simulink model "SatDinModel_3_TES_RW_OL"  (Simulink 7.7)
settings: Solver=ode45  StartTime=0.0  StopTime=40  FixedStep=1  RelTol=1e-3
undefined symbols (not defined in the file or in its folder): coe2rv, e0_0, e1_0, e2_0, e3_0, pm_0, rv2OrbFrame, sigbuilder_block, Vm_0, xme_0
libraries: aerolibtransform2 x8, aerolibconvert2 x8, aerolibutil x3, simulink x2, aerolibanimutils x1, aerolibanim x1, vrlib x1
settings Model: Creator=Ridanto  LastModifiedBy=Ridanto  BufferReuse=off
settings OptimizationCC: BufferReuse=off  InitFltsAndDblsToZero=on
settings DebuggingCC: SaveWithParameterizedLinksMsg=none  SignalResolutionControl=TryResolveAllWithWarning  MultiTaskDSMMsg=warning  MultiTaskCondExecSysMsg=none  StrictBusMsg=Warning
settings SFSimCC: SimParseCustomCode=off
settings RTWCC: IncludeERTFirstTime=on
settings GRTTargetCC: TargetFcnLib=ansi_tfl_tmw.mat

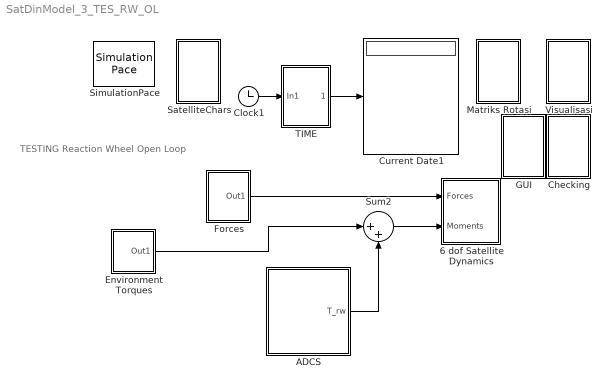
== system SatDinModel_3_TES_RW_OL ==
  note: TESTING
      | Reaction Wheel Open Loop
  6 dof Satellite Dynamics : Subsystem
  ADCS : Subsystem
  Checking : Subsystem
  Clock1 : Clock
      settings: Decimation=10
  Current Date1 : Display
  Environment Torques : Subsystem
  Forces : Subsystem
  GUI : Subsystem
  Matriks Rotasi : Subsystem
  SatelliteChars : Subsystem
  SimulationPace : aerolibanimutils/Simulation Pace  SimulationPace=60  SleepMode=MATLAB Thread  OutputPaceError=off  SampleTime=1/30
      settings: AttributesFormatString=%<SimulationPace> sec/sec
  Sum2 : Sum  Inputs=|++
  TIME : Subsystem
  Visualisasi : Subsystem
  wires:
  Clock1/1 -> TIME/1(In1)
  TIME/1(Out1) -> Current Date1/1
  Environment Torques/1(Out1) -> Sum2/1
  Sum2/1 -> 6 dof Satellite Dynamics/2(Moments)
  Forces/1(Out1) -> 6 dof Satellite Dynamics/1(Forces)
  ADCS/1(T_rw) -> Sum2/2

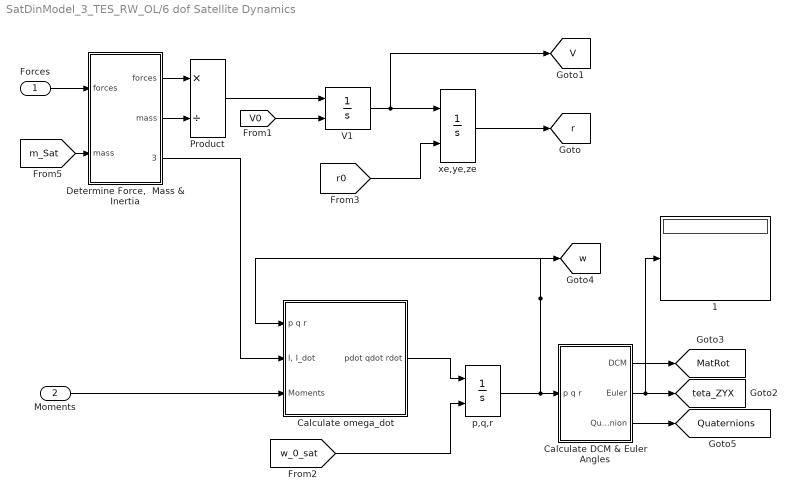
== system SatDinModel_3_TES_RW_OL/6 dof Satellite Dynamics ==
  Forces : Inport
  Moments : Inport  Port=2
  1 : Display
  Calculate DCM & Euler Angles : Subsystem  AncestorBlock=aerolib6dofsys/DCM & Euler Angles (Quaternion)
      mask Type: DCM & Euler Angles (Quaternion)
  Calculate omega_dot : Subsystem  AncestorBlock=aerolib6dofsys/Calculate omega_dot
  "Determine Force,  Mass & Inertia" : Subsystem  AncestorBlock=aerolib6dofsys/Mass & Inertia (fixed)
      mask Type: Mass & Inertia (fixed)
  Product : Product  Inputs=*/  SaturateOnIntegerOverflow=on  OutDataTypeStr=Inherit: Same as first input
  V1 : Integrator  InitialConditionSource=external  InitialCondition=convvel(Vm_0,'m/s','m/s')
  "p,q,r " : Integrator  InitialConditionSource=external  InitialCondition=pm_0
  xe,ye,ze : Integrator  InitialConditionSource=external  InitialCondition=xme_0
  tag scope: MatRot=global, Quaternions=global, V=global, r=global, teta_ZYX=global, w=global
  wires:
  "Determine Force,  Mass & Inertia"/1("forces ") -> Product/1
  Calculate omega_dot/1(pdot qdot rdot) -> "p,q,r "/1
  "Determine Force,  Mass & Inertia"/2(mass) -> Product/2
  Calculate DCM & Euler Angles/1(DCM) -> [MatRot]
  Product/1 -> V1/1
  Forces/1 -> "Determine Force,  Mass & Inertia"/1(forces)
  Moments/1 -> Calculate omega_dot/3(Moments)
  "p,q,r "/1 -> Calculate omega_dot/1(p q r), Calculate DCM & Euler Angles/1(p q r), [w]
  xe,ye,ze/1 -> [r]
  Calculate DCM & Euler Angles/2(Euler) -> [teta_ZYX], 1/1
  "Determine Force,  Mass & Inertia"/3("inertia, 0") -> Calculate omega_dot/2("I, I_dot")
  [w_0_sat] -> "p,q,r "/2
  [r0] -> xe,ye,ze/2
  Calculate DCM & Euler Angles/3(Quaternion) -> [Quaternions]
  [m_Sat] -> "Determine Force,  Mass & Inertia"/2("mass ")
  [V0] -> V1/2
  V1/1 -> xe,ye,ze/1, [V]

== system SatDinModel_3_TES_RW_OL/ADCS ==
  Mux : Mux  Inputs=3
  RW_3_Axis : Subsystem
  Signal Builder : Subsystem  Tag=STV Subsys  LoadFcn=sigbuilder_block('load');  StartFcn=sigbuilder_block('start');  StopFcn=sigbuilder_block('stop');  ClipboardFcn=sigbuilder_block('clipboard');  mask(Sigbuilder block){}
      mask help: Create and generate interchangeable groups of signals whose waveforms are piecewise linear.
      mask init:
      | if ~strcmp(get_param(bdroot(gcbh),'SimulationStatus'),'stopped') tuvar = sigbuilder_block('maskInit'); end
      settings: CopyFcn=sigbuilder_block('copy');  DeleteFcn=sigbuilder_block('delete');  ModelCloseFcn=sigbuilder_block('modelClose');  PreSaveFcn=sigbuilder_block('preSave');  NameChangeFcn=sigbuilder_block('namechange');  OpenFcn=sigbuilder_block('open',[437.25 96 550.5 394.5 ]);  CloseFcn=sigbuilder_block('close');
      mask Display: plot(0, 0, 100, 100,[2, 2, 32, 32, 2], [68, 8, 8, 68, 68],[32, 2], [38, 38], [32, 19, 2],[53, 60, 44], [32, 17, 17, 2],[16, 16, 31, 31]);txt = getActiveGroup(gcbh);text(2, 100, txt,'verticalAlignment', 'top');
  w_rw : Scope
      settings: SaveName=ScopeData6
  T_rw : Outport
  tag scope: H_rw=global, w_rw=global
  wires:
  RW_3_Axis/1(T_rw) -> T_rw/1
  RW_3_Axis/2(w_rw) -> [w_rw], w_rw/1
  RW_3_Axis/3(H_rw) -> [H_rw]
  Mux/1 -> RW_3_Axis/1(T_c)
  Signal Builder/1(Signal 1) -> Mux/1
  Signal Builder/2(Signal 5) -> Mux/2
  Signal Builder/3(Signal 6) -> Mux/3

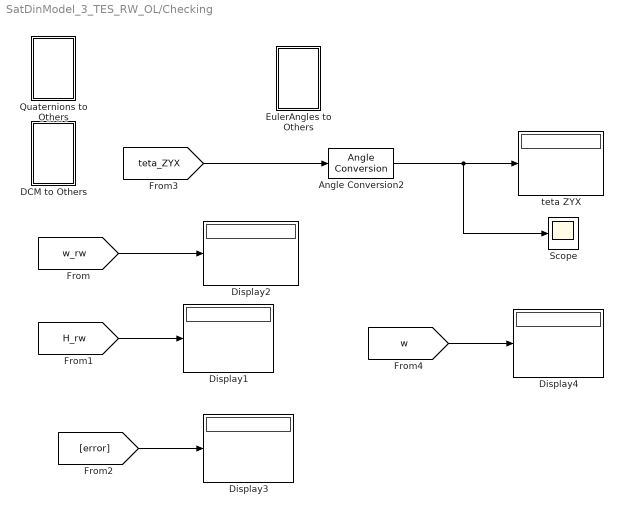
== system SatDinModel_3_TES_RW_OL/Checking ==
  Angle Conversion2 : aerolibconvert2/Angle Conversion  SystemSampleTime=-1  IU=rad  OU=deg
  DCM to Others : Subsystem
  Display{1..4} (4 alike) : Display
  EulerAngles to Others : Subsystem
  Quaternions to Others : Subsystem
  Scope : Scope
      settings: YMin=0  YMax=0.00275
  teta ZYX : Display
  wires:
  [H_rw] -> Display1/1
  [w_rw] -> Display2/1
  [error] -> Display3/1
  [teta_ZYX] -> Angle Conversion2/1
  [w] -> Display4/1
  Angle Conversion2/1 -> teta ZYX/1, Scope/1

== system SatDinModel_3_TES_RW_OL/Environment Torques ==
  "Env Torque, Nm" : Subsystem  Tag=STV Subsys  LoadFcn=sigbuilder_block('load');  StartFcn=sigbuilder_block('start');  StopFcn=sigbuilder_block('stop');  ClipboardFcn=sigbuilder_block('clipboard');  mask(Sigbuilder block){}
      mask help: Create and generate interchangeable groups of signals whose waveforms are piecewise linear.
      mask init:
      | if ~strcmp(get_param(bdroot(gcbh),'SimulationStatus'),'stopped') tuvar = sigbuilder_block('maskInit'); end
      settings: CopyFcn=sigbuilder_block('copy');  DeleteFcn=sigbuilder_block('delete');  ModelCloseFcn=sigbuilder_block('modelClose');  PreSaveFcn=sigbuilder_block('preSave');  NameChangeFcn=sigbuilder_block('namechange');  OpenFcn=sigbuilder_block('open',[437.25 96 550.5 394.5 ]);  CloseFcn=sigbuilder_block('close');
      mask Display: plot(0,0,100,100,[10,10,40,40,10],[80,20,20,80,80],[40,10],[50,50], [40,27,10],[65,72,56],[40,25,25,10],[28,28,43,43]);
  Manual Switch : simulink/Signal Routing/Manual Switch  SystemSampleTime=-1  sw=1  action=0  varsize=off
  Mux : Mux  Inputs=3
  No Torque : Constant  Value=[0 0 0]
  Typical LEO SSO : Gain  Gain=4.586e-5
  xxx : Constant  Value=0
  Out1 : Outport
  wires:
  xxx/1 -> Mux/2, Mux/3
  Mux/1 -> Manual Switch/2
  No Torque/1 -> Manual Switch/1
  Manual Switch/1 -> Out1/1
  "Env Torque, Nm"/1(Signal 1) -> Typical LEO SSO/1
  Typical LEO SSO/1 -> Mux/1

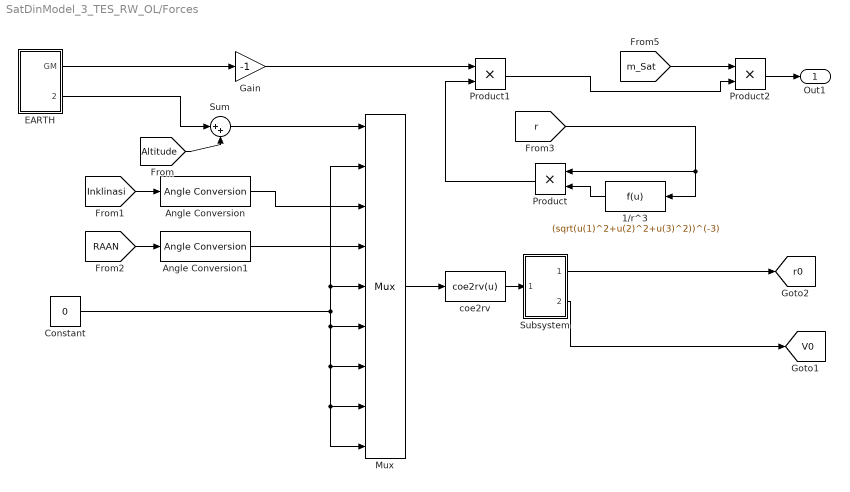
== system SatDinModel_3_TES_RW_OL/Forces ==
  1/r^3 : Fcn  Expr=(sqrt(u(1)^2+u(2)^2+u(3)^2))^(-3)
  Angle Conversion : aerolibconvert2/Angle Conversion  SystemSampleTime=-1  IU=deg  OU=rad
  Angle Conversion1 : aerolibconvert2/Angle Conversion  SystemSampleTime=-1  IU=deg  OU=rad
  Constant : Constant  Value=0
  EARTH : Subsystem
  Gain : Gain  Gain=-1
  Mux : Mux  Inputs=9
  Product : Product  RndMeth=Zero
  Product1 : Product  RndMeth=Zero
  Product2 : Product  RndMeth=Zero
  Subsystem : Subsystem
  Sum : Sum  Inputs=|++
  coe2rv : MATLABFcn  MATLABFcn=coe2rv(u)
  Out1 : Outport
  tag scope: V0=global, r0=global
  wires:
  EARTH/1(GM) -> Gain/1
  EARTH/2(Radius) -> Sum/1
  Angle Conversion/1 -> Mux/3
  Sum/1 -> Mux/1
  Angle Conversion1/1 -> Mux/4
  Mux/1 -> coe2rv/1
  coe2rv/1 -> Subsystem/1(In1)
  Constant/1 -> Mux/2, Mux/5, Mux/6, Mux/7, Mux/8, Mux/9
  [Altitude] -> Sum/2
  [Inklinasi] -> Angle Conversion/1
  [RAAN] -> Angle Conversion1/1
  Subsystem/1(Out1) -> [r0]
  1/r^3/1 -> Product/2
  Product/1 -> Product1/2
  Gain/1 -> Product1/1
  Product1/1 -> Product2/2
  [r] -> 1/r^3/1, Product/1
  [m_Sat] -> Product2/1
  Product2/1 -> Out1/1
  Subsystem/2(Out2) -> [V0]

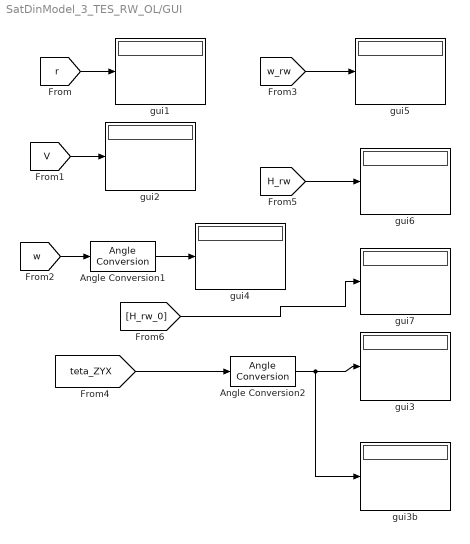
== system SatDinModel_3_TES_RW_OL/GUI ==
  Angle Conversion1 : aerolibconvert2/Angle Conversion  SystemSampleTime=-1  IU=rad  OU=deg
  Angle Conversion2 : aerolibconvert2/Angle Conversion  SystemSampleTime=-1  IU=rad  OU=deg
  gui{1..7} (7 alike) : Display
  gui3b : Display
  wires:
  [r] -> gui1/1
  [V] -> gui2/1
  Angle Conversion1/1 -> gui4/1
  [w] -> Angle Conversion1/1
  [teta_ZYX] -> Angle Conversion2/1
  Angle Conversion2/1 -> gui3/1, gui3b/1
  [w_rw] -> gui5/1
  [H_rw] -> gui6/1
  [H_rw_0] -> gui7/1

== system SatDinModel_3_TES_RW_OL/Matriks Rotasi ==
  Math Function : Math  Operator=transpose  SaturateOnIntegerOverflow=on
  Matriks Rotasi Benda-Inersial : Display
  Matriks Rotasi Benda-Orbital : Display
  Matriks Rotasi Orbital-Inersial : Display
  Mux1 : Mux  Inputs=2
  Product : Product  Multiplication=Matrix(*)  RndMeth=Zero
  rv2OrbFrame : MATLABFcn  MATLABFcn=rv2OrbFrame(u)  Output1D=off
  tag scope: R_oi=global
  wires:
  [r] -> Mux1/1
  [V] -> Mux1/2
  Mux1/1 -> rv2OrbFrame/1
  rv2OrbFrame/1 -> Matriks Rotasi Orbital-Inersial/1, Math Function/1, [R_oi]
  [MatRot] -> Matriks Rotasi Benda-Inersial/1, Product/1
  Math Function/1 -> Product/2
  Product/1 -> Matriks Rotasi Benda-Orbital/1

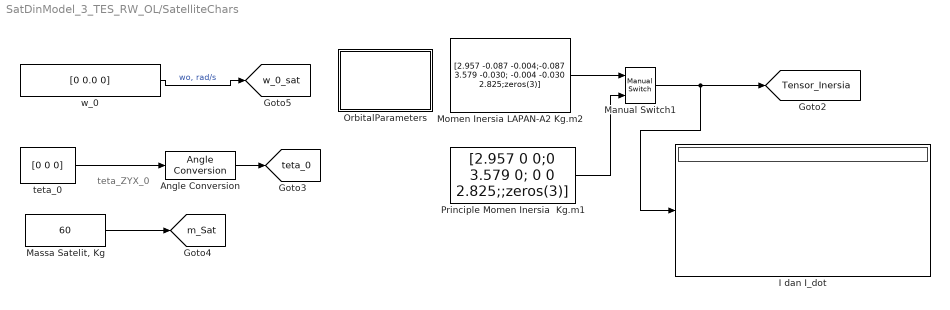
== system SatDinModel_3_TES_RW_OL/SatelliteChars ==
  note: teta_ZYX_0
  Angle Conversion : aerolibconvert2/Angle Conversion  SystemSampleTime=-1  IU=deg  OU=rad
  I dan I_dot : Display
  Manual Switch1 : simulink/Signal Routing/Manual Switch  SystemSampleTime=-1  sw=1  action=0  varsize=off
  "Massa Satelit, Kg" : Constant  Value=60
  Momen Inersia LAPAN-A2 Kg.m2 : Constant  Value=[2.957 -0.087 -0.004;-0.087 3.579 -0.030; -0.004 -0.030 2.825;zeros(3)]
  OrbitalParameters : Subsystem
  Principle Momen Inersia  Kg.m1 : Constant  Value=[2.957 0 0;0 3.579 0; 0 0 2.825;;zeros(3)]
  teta_0 : Constant  Value=[0 0 0]
  w_0 : Constant  Value=[0 0.0 0]
  tag scope: Tensor_Inersia=global, m_Sat=global, teta_0=global, w_0_sat=global
  wires:
  teta_0/1 -> Angle Conversion/1
  "Massa Satelit, Kg"/1 -> [m_Sat]
  Angle Conversion/1 -> [teta_0]
  Principle Momen Inersia  Kg.m1/1 -> Manual Switch1/2
  Momen Inersia LAPAN-A2 Kg.m2/1 -> Manual Switch1/1
  Manual Switch1/1 -> [Tensor_Inersia], I dan I_dot/1
  w_0/1 -> [w_0_sat]  "wo, rad/s"

== system SatDinModel_3_TES_RW_OL/TIME ==
  In1 : Inport
  Embedded MATLAB Function : Stateflow chart  TreatAsAtomicUnit=on
  JD : Display
  Sum1 : Sum  Inputs=|++
  day2second : Gain  Gain=1/3600/24
  detik : Display
  Out1 : Outport
  wires:
  In1/1 -> detik/1, day2second/1
  day2second/1 -> Sum1/1
  Sum1/1 -> Embedded MATLAB Function/1(jd), JD/1
  Embedded MATLAB Function/1(y) -> Out1/1
  [Mulai] -> Sum1/2

== system SatDinModel_3_TES_RW_OL/Visualisasi ==
  6DoF Animation : aerolibanim/6DoF Animation  SystemSampleTime=-1  u1=[-10000 10000 -10000 10000 -10000 10000]  u2=2  u3=2000  u4=[0 0 0]  u5=Fixed position  u6=[60000 120000 60000]  u7=10  u8=on
      link override Animation S-Function: FunctionName=sSATanim3
  Display : Display
  Gain : Gain  Gain=1/500
  Selector : Selector  InputPortWidth=3  IndexOptions=Index vector (dialog)  Indices=[3 2 1]  OutputSizes=1
  VR Sink1 : vrlib/VR Sink  SampleTime=20  ViewEnable=on  RemoteChange=off  RemoteView=on  FieldsWritten=satelit.rotation.4.1.1.double#satelit.translation.3.1.1.double  WorldFileName=vrattsat.WRL  AutoView=off  VideoDimensions=[]  FigureProperties={}
  wires:
  [teta_ZYX] -> Selector/1
  [r] -> 6DoF Animation/1, Display/1, Gain/1
  Selector/1 -> 6DoF Animation/2
  [Quaternions] -> VR Sink1/1
  Gain/1 -> VR Sink1/2

== system SatDinModel_3_TES_RW_OL/6 dof Satellite Dynamics/Calculate DCM & Euler Angles ==
  p q r : Inport
  Quaternions to  Direction Cosine Matrix : aerolibtransform2/Quaternions to  Direction Cosine Matrix  SystemSampleTime=-1
  Quaternions to Rotation Angles : aerolibtransform2/Quaternions to Rotation Angles  SystemSampleTime=-1  rotationOrder=ZYX
  Rotation Angles to Quaternions : aerolibtransform2/Rotation Angles to Quaternions  SystemSampleTime=-1  rotationOrder=ZYX
  q0 q1 q2 q3 : Integrator  InitialConditionSource=external  InitialCondition=[e0_0 e1_0 e2_0 e3_0]
  qdot : Subsystem
  DCM : Outport
  Euler : Outport  Port=2
  Quaternion : Outport  Port=3
  wires:
  Quaternions to Rotation Angles/1 -> Euler/1
  Quaternions to  Direction Cosine Matrix/1 -> DCM/1
  p q r/1 -> qdot/1(p q r)
  [teta_0] -> Rotation Angles to Quaternions/1
  Rotation Angles to Quaternions/1 -> q0 q1 q2 q3/2
  q0 q1 q2 q3/1 -> Quaternions to Rotation Angles/1, qdot/2(q0 q1 q2 q3), Quaternions to  Direction Cosine Matrix/1, Quaternion/1
  qdot/1(qdot) -> q0 q1 q2 q3/1

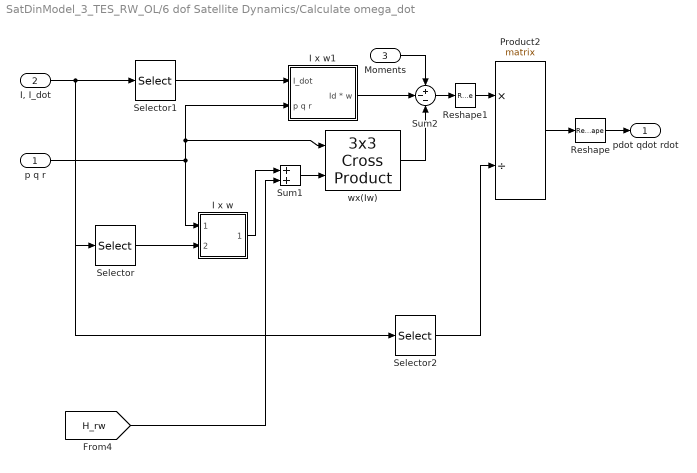
== system SatDinModel_3_TES_RW_OL/6 dof Satellite Dynamics/Calculate omega_dot ==
  p q r : Inport
  "I, I_dot" : Inport  Port=2
  Moments : Inport  Port=3
  I x w : Subsystem
  I x w1 : Subsystem
  Product2 : Product  Inputs=*/  Multiplication=Matrix(*)  SaturateOnIntegerOverflow=on  OutDataTypeStr=Inherit: Same as first input
  Reshape : Reshape
  Reshape1 : Reshape  OutputDimensionality=Row vector (2-D)
  Selector : Selector  NumberOfDimensions=2  InputPortWidth=2  IndexOptions=Index vector (dialog),Select all  Indices=1:3,-1  OutputSizes=1
  Selector1 : Selector  NumberOfDimensions=2  InputPortWidth=2  IndexOptions=Index vector (dialog),Select all  Indices=4:6,-1  OutputSizes=1
  Selector2 : Selector  NumberOfDimensions=2  InputPortWidth=2  IndexOptions=Index vector (dialog),Select all  Indices=1:3,-1  OutputSizes=1
  Sum1 : Sum  SaturateOnIntegerOverflow=on
  Sum2 : Sum  Inputs=+--  SaturateOnIntegerOverflow=on
  wx(Iw) : aerolibutil/3x3 Cross Product  SystemSampleTime=-1
  pdot qdot rdot : Outport
  wires:
  Reshape1/1 -> Product2/1
  wx(Iw)/1 -> Sum2/3
  Selector1/1 -> I x w1/1(I_dot)
  I x w1/1(Id * w) -> Sum2/2
  Moments/1 -> Sum2/1
  Sum2/1 -> Reshape1/1
  Product2/1 -> Reshape/1
  p q r/1 -> I x w1/2(p q r), wx(Iw)/1, I x w/1(p q r)
  "I, I_dot"/1 -> Selector1/1, Selector2/1, Selector/1
  Selector2/1 -> Product2/2
  Selector/1 -> I x w/2(Inertia)
  Reshape/1 -> pdot qdot rdot/1
  Sum1/1 -> wx(Iw)/2
  I x w/1(I * w) -> Sum1/1
  [H_rw] -> Sum1/2

== system SatDinModel_3_TES_RW_OL/6 dof Satellite Dynamics/Determine Force,  Mass & Inertia ==
  forces : Inport
  "mass " : Inport  Port=2
  "forces " : Outport
  mass : Outport  Port=2
  "inertia, 0" : Outport  Port=3
  wires:
  forces/1 -> "forces "/1
  [Tensor_Inersia] -> "inertia, 0"/1
  "mass "/1 -> mass/1

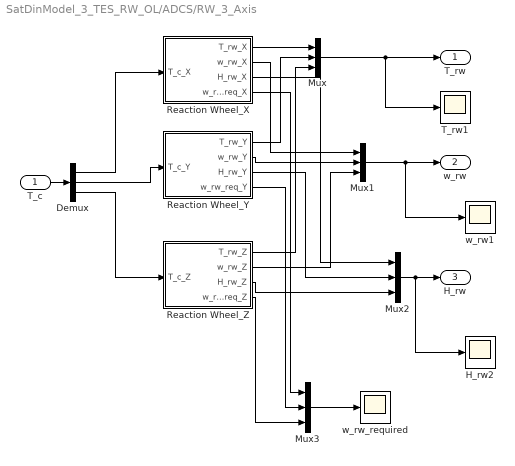
== system SatDinModel_3_TES_RW_OL/ADCS/RW_3_Axis ==
  T_c : Inport
  Demux : Demux  Outputs=3
  H_rw2 : Scope
      settings: SaveName=ScopeData3
  Mux{,1..3} (4 alike) : Mux  Inputs=3
  Reaction Wheel_X : Subsystem
  Reaction Wheel_Y : Subsystem
  Reaction Wheel_Z : Subsystem
  T_rw1 : Scope
      settings: SaveName=ScopeData10
  w_rw1 : Scope
  w_rw_required : Scope
      settings: SaveName=ScopeData2
  T_rw : Outport
  w_rw : Outport  Port=2
  H_rw : Outport  Port=3
  wires:
  Reaction Wheel_Y/1(T_rw_Y) -> Mux/2
  T_c/1 -> Demux/1
  Demux/1 -> Reaction Wheel_X/1(T_c_X)
  Demux/2 -> Reaction Wheel_Y/1(T_c_Y)
  Demux/3 -> Reaction Wheel_Z/1(T_c_Z)
  Reaction Wheel_X/1(T_rw_X) -> Mux/1
  Reaction Wheel_Z/1(T_rw_Z) -> Mux/3
  Mux/1 -> T_rw/1, T_rw1/1
  Mux1/1 -> w_rw/1, w_rw1/1
  Reaction Wheel_Y/2(w_rw_Y) -> Mux1/2
  Reaction Wheel_X/2(w_rw_X) -> Mux1/1
  Reaction Wheel_Z/2(w_rw_Z) -> Mux1/3
  Mux2/1 -> H_rw/1, H_rw2/1
  Reaction Wheel_Z/3(H_rw_Z) -> Mux2/3
  Reaction Wheel_X/3(H_rw_X) -> Mux2/1
  Reaction Wheel_Y/3(H_rw_Y) -> Mux2/2
  Mux3/1 -> w_rw_required/1
  Reaction Wheel_X/4(w_rw_req_X) -> Mux3/1
  Reaction Wheel_Y/4(w_rw_req_Y) -> Mux3/2
  Reaction Wheel_Z/4(w_rw_req_Z) -> Mux3/3

== system SatDinModel_3_TES_RW_OL/ADCS/Signal Builder ==
  Demux : Demux  Tag=STV Demux  Outputs=3
  FromWs : FromWorkspace  Tag=STV FromWs  VariableName=tuvar  SampleTime=0  SigBuilderData=DataTag0  VnvData=DataTag1
      SigBuilderData=|
      | common.afterFinalStr = 'Extrapolate'
      | common.sampleTime = 0
      | dataSet.timeRange = [0 10]
      | dataSet.name = 'Group 1'
      | sbobj.Groups.Name = 'Group 1'
      | sbobj.Groups.Signals(1).Name = 'Signal 1'
      | sbobj.Groups.Signals(1).XData = [0 4 4 5.04 5.04 10]
      | sbobj.Groups.Signals(1).YData = [0 0 0.1 0.1 0 0]
      | sbobj.Groups.Signals(2).Name = 'Signal 5'
      | sbobj.Groups.Signals(2).XData = [0 4 4 6 6 10]
      | sbobj.Groups.Signals(2).YData = [0 0 0.1 0.1 0 0]
      | sbobj.Groups.Signals(3).Name = 'Signal 6'
      | sbobj.Groups.Signals(3).XData = [0 5 5 7 7 10]
      | sbobj.Groups.Signals(3).YData = [0 0 0.062 0.062 0 0]
  Signal 1 : Outport  Tag=STV Outport
  Signal 5 : Outport  Tag=STV Outport  Port=2
  Signal 6 : Outport  Tag=STV Outport  Port=3
  wires:
  Demux/1 -> Signal 1/1
  FromWs/1 -> Demux/1
  Demux/2 -> Signal 5/1
  Demux/3 -> Signal 6/1

== system SatDinModel_3_TES_RW_OL/Checking/DCM to Others ==
  Angle Conversion : aerolibconvert2/Angle Conversion  SystemSampleTime=-1  IU=rad  OU=deg
  Direction Cosine Matrix  to Quaternions : aerolibtransform2/Direction Cosine Matrix  to Quaternions  SystemSampleTime=-1
  "Quaternions q0, q1, q2, q3" : Display
  Quaternions to Rotation Angles : aerolibtransform2/Quaternions to Rotation Angles  SystemSampleTime=-1  rotationOrder=ZYX
  teta_Euler ZYX : Display
  "teta_Euler ZYX " : Display
  wires:
  Quaternions to Rotation Angles/1 -> teta_Euler ZYX/1, Angle Conversion/1
  Angle Conversion/1 -> "teta_Euler ZYX "/1
  [MatRot] -> Direction Cosine Matrix  to Quaternions/1
  Direction Cosine Matrix  to Quaternions/1 -> "Quaternions q0, q1, q2, q3"/1, Quaternions to Rotation Angles/1

== system SatDinModel_3_TES_RW_OL/Checking/EulerAngles to Others ==
  Direction Cosine Matrix  to Quaternions : aerolibtransform2/Direction Cosine Matrix  to Quaternions  SystemSampleTime=-1
  Matriks Rotasi Benda-Inersial R_bi : Display
  "Quaternions q0, q1, q2, q3" : Display
  teta_ZYX to DCM : Subsystem
  wires:
  [teta_ZYX] -> teta_ZYX to DCM/1(In2)
  Direction Cosine Matrix  to Quaternions/1 -> "Quaternions q0, q1, q2, q3"/1
  teta_ZYX to DCM/1(Out1) -> Matriks Rotasi Benda-Inersial R_bi/1, Direction Cosine Matrix  to Quaternions/1

== system SatDinModel_3_TES_RW_OL/Checking/Quaternions to Others ==
  Angle Conversion : aerolibconvert2/Angle Conversion  SystemSampleTime=-1  IU=rad  OU=deg
  Matriks Rotasi Benda-Inersial R_bi : Display
  Matriks Rotasi Benda-Inersial R_bi _juga : Display
  Quaternions to  Direction Cosine Matrix : aerolibtransform2/Quaternions to  Direction Cosine Matrix  SystemSampleTime=-1
  Quaternions to Rotation Angles : aerolibtransform2/Quaternions to Rotation Angles  SystemSampleTime=-1  rotationOrder=ZYX
  teta_Euler ZYX : Display
  "teta_Euler ZYX " : Display
  teta_ZYX to DCM : Subsystem
  wires:
  Quaternions to Rotation Angles/1 -> teta_Euler ZYX/1, Angle Conversion/1, teta_ZYX to DCM/1(In2)
  teta_ZYX to DCM/1(Out1) -> Matriks Rotasi Benda-Inersial R_bi/1
  Quaternions to  Direction Cosine Matrix/1 -> Matriks Rotasi Benda-Inersial R_bi _juga/1
  Angle Conversion/1 -> "teta_Euler ZYX "/1
  [Quaternions] -> Quaternions to Rotation Angles/1, Quaternions to  Direction Cosine Matrix/1

== system SatDinModel_3_TES_RW_OL/Environment Torques/Env Torque, Nm ==
  Demux : Demux  Tag=STV Demux  Outputs=1
  FromWs : FromWorkspace  Tag=STV FromWs  VariableName=tuvar  SampleTime=0  SigBuilderData=DataTag2  VnvData=DataTag3
      SigBuilderData=|
      | common.afterFinalStr = 'Extrapolate'
      | common.sampleTime = 0
      | dataSet.timeRange = [0 10]
      | dataSet.name = 'Group 1'
      | sbobj.Groups.Name = 'Group 1'
      | sbobj.Groups.Signals.Name = 'Signal 1'
      | sbobj.Groups.Signals.XData = [0 4 4 6 6 10]
      | sbobj.Groups.Signals.YData = [0 0 1 1 0 0]
  Signal 1 : Outport  Tag=STV Outport
  wires:
  Demux/1 -> Signal 1/1
  FromWs/1 -> Demux/1

== system SatDinModel_3_TES_RW_OL/Forces/EARTH ==
  GM Earth : Constant  Value=3.986e5
  Re : Constant  Value=6378
  GM : Outport
  Radius : Outport  Port=2
  wires:
  GM Earth/1 -> GM/1
  Re/1 -> Radius/1

== system SatDinModel_3_TES_RW_OL/Forces/Subsystem ==
  In1 : Inport
  Demux : Demux  Outputs=6
  Mux1 : Mux  Inputs=3
  Mux2 : Mux  Inputs=3
  Out1 : Outport
  Out2 : Outport  Port=2
  wires:
  Demux/1 -> Mux1/1
  Demux/2 -> Mux1/2
  Demux/3 -> Mux1/3
  Demux/4 -> Mux2/1
  Demux/5 -> Mux2/2
  Demux/6 -> Mux2/3
  Mux1/1 -> Out1/1
  In1/1 -> Demux/1
  Mux2/1 -> Out2/1

== system SatDinModel_3_TES_RW_OL/SatelliteChars/OrbitalParameters ==
  Epoch : Constant  Value=735578.8723
  H : Constant  Value=800
  Inclination : Constant  Value=98.7192
  RAAN : Constant  Value=86.1494
  tag scope: Altitude=global, Inklinasi=global, Mulai=global, RAAN=global
  wires:
  H/1 -> [Altitude]
  Inclination/1 -> [Inklinasi]
  RAAN/1 -> [RAAN]
  Epoch/1 -> [Mulai]

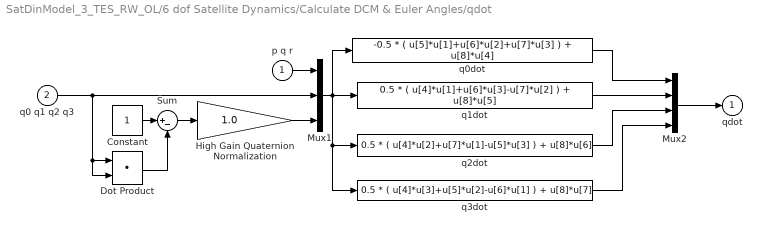
== system SatDinModel_3_TES_RW_OL/6 dof Satellite Dynamics/Calculate DCM & Euler Angles/qdot ==
  p q r : Inport
  q0 q1 q2 q3 : Inport  Port=2
  Constant : Constant
  Dot Product : DotProduct  OutDataTypeStr=Inherit: Inherit via internal rule
  High Gain Quaternion Normalization : Gain  Gain=1.0  SaturateOnIntegerOverflow=on  OutDataTypeStr=Inherit: Same as input  ParamDataTypeStr=Inherit: Same as input
  Mux1 : Mux  Inputs=[3 4 1]
  Mux2 : Mux
  Sum : Sum  Inputs=|+-  SaturateOnIntegerOverflow=on  InputSameDT=on  OutDataTypeStr=Inherit: Same as first input
  q0dot : Fcn  Expr=-0.5 * ( u[5]*u[1]+u[6]*u[2]+u[7]*u[3] ) + u[8]*u[4]
  q1dot : Fcn  Expr=0.5 * ( u[4]*u[1]+u[6]*u[3]-u[7]*u[2] ) + u[8]*u[5]
  q2dot : Fcn  Expr=0.5 * ( u[4]*u[2]+u[7]*u[1]-u[5]*u[3] ) + u[8]*u[6]
  q3dot : Fcn  Expr=0.5 * ( u[4]*u[3]+u[5]*u[2]-u[6]*u[1] ) + u[8]*u[7]
  qdot : Outport  InitialOutput=0
  wires:
  p q r/1 -> Mux1/1
  Dot Product/1 -> Sum/2
  High Gain Quaternion Normalization/1 -> Mux1/3
  Sum/1 -> High Gain Quaternion Normalization/1
  Constant/1 -> Sum/1
  Mux2/1 -> qdot/1
  q0dot/1 -> Mux2/1
  q1dot/1 -> Mux2/2
  q2dot/1 -> Mux2/3
  Mux1/1 -> q2dot/1, q3dot/1, q0dot/1, q1dot/1
  q3dot/1 -> Mux2/4
  q0 q1 q2 q3/1 -> Dot Product/1, Dot Product/2, Mux1/2

== system SatDinModel_3_TES_RW_OL/6 dof Satellite Dynamics/Calculate omega_dot/I x w ==
  p q r : Inport
  Inertia : Inport  Port=2
  Product : Product  Multiplication=Matrix(*)  SaturateOnIntegerOverflow=on  InputSameDT=on  OutDataTypeStr=Inherit: Same as first input
  Reshape1 : Reshape  OutputDimensionality=Column vector (2-D)
  Reshape2 : Reshape
  I * w : Outport
  wires:
  Reshape2/1 -> I * w/1
  Reshape1/1 -> Product/2
  p q r/1 -> Reshape1/1
  Inertia/1 -> Product/1
  Product/1 -> Reshape2/1

== system SatDinModel_3_TES_RW_OL/6 dof Satellite Dynamics/Calculate omega_dot/I x w1 ==
  I_dot : Inport
  p q r : Inport  Port=2
  Product : Product  Multiplication=Matrix(*)  SaturateOnIntegerOverflow=on  InputSameDT=on  OutDataTypeStr=Inherit: Same as first input
  Reshape1 : Reshape  OutputDimensionality=Column vector (2-D)
  Reshape2 : Reshape
  Id * w : Outport
  wires:
  Reshape2/1 -> Id * w/1
  Reshape1/1 -> Product/2
  Product/1 -> Reshape2/1
  I_dot/1 -> Product/1
  p q r/1 -> Reshape1/1

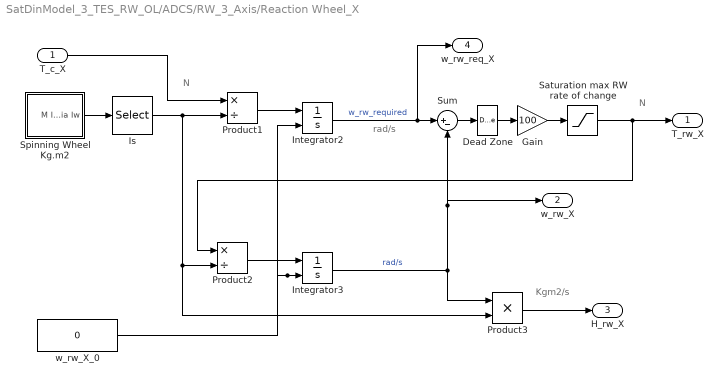
== system SatDinModel_3_TES_RW_OL/ADCS/RW_3_Axis/Reaction Wheel_X ==
  note: rad/s
  note: N
  note: N
  note: Kgm2/s
  T_c_X : Inport
  Dead Zone : DeadZone  SaturateOnIntegerOverflow=on
  Gain : Gain  Gain=100
  Integrator2 : Integrator  InitialConditionSource=external
  Integrator3 : Integrator  InitialConditionSource=external
  Is : Selector  InputPortWidth=3  IndexOptions=Index vector (dialog)  Indices=[1]  OutputSizes=1
  Product1 : Product  Inputs=*/  RndMeth=Zero
  Product2 : Product  Inputs=*/  RndMeth=Zero
  Product3 : Product  RndMeth=Zero
  "Saturation max RW rate of change " : Saturate  UpperLimit=0.0075  LowerLimit=-0.0075
  Spinning Wheel Kg.m2 : Subsystem  mask{D=0.1, t=0.01, rho=5000}
      mask prompts: D "diameter"; t "tebal"; rho "density"
  Sum : Sum  Inputs=|+-
  w_rw_X_0 : Constant  Value=0
  T_rw_X : Outport
  w_rw_X : Outport  Port=2
  H_rw_X : Outport  Port=3
  w_rw_req_X : Outport  Port=4
  wires:
  T_c_X/1 -> Product1/1
  Is/1 -> Product1/2, Product2/2, Product3/2
  Product1/1 -> Integrator2/1
  w_rw_X_0/1 -> Integrator2/2, Integrator3/2
  Integrator2/1 -> Sum/1, w_rw_req_X/1  "w_rw_required"
  Integrator3/1 -> Sum/2, w_rw_X/1, Product3/1  "rad/s"
  Sum/1 -> Dead Zone/1
  Gain/1 -> "Saturation max RW rate of change "/1
  Product2/1 -> Integrator3/1
  "Saturation max RW rate of change "/1 -> Product2/1, T_rw_X/1
  Spinning Wheel Kg.m2/1(M Inertia Iw) -> Is/1
  Product3/1 -> H_rw_X/1
  Dead Zone/1 -> Gain/1

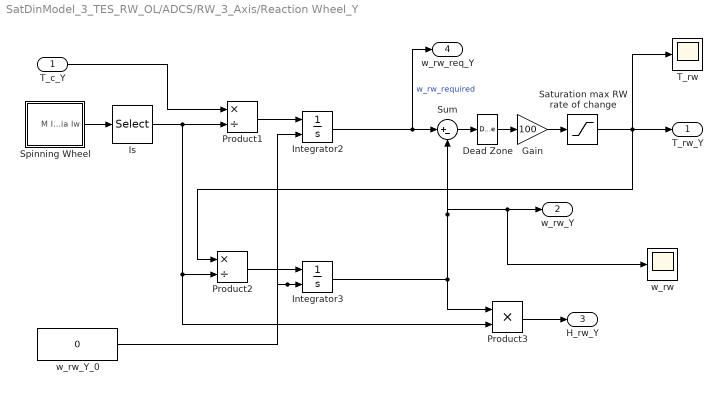
== system SatDinModel_3_TES_RW_OL/ADCS/RW_3_Axis/Reaction Wheel_Y ==
  T_c_Y : Inport
  Dead Zone : DeadZone  SaturateOnIntegerOverflow=on
  Gain : Gain  Gain=100
  Integrator2 : Integrator  InitialConditionSource=external
  Integrator3 : Integrator  InitialConditionSource=external
  Is : Selector  InputPortWidth=3  IndexOptions=Index vector (dialog)  Indices=[1]  OutputSizes=1
  Product1 : Product  Inputs=*/  RndMeth=Zero
  Product2 : Product  Inputs=*/  RndMeth=Zero
  Product3 : Product  RndMeth=Zero
  "Saturation max RW rate of change " : Saturate  UpperLimit=0.0075  LowerLimit=-0.0075
  Spinning Wheel : Subsystem  mask{D=0.1, t=0.01, rho=2850}
      mask prompts: D "diameter"; t "tebal"; rho "density"
  Sum : Sum  Inputs=|+-
  T_rw : Scope
      settings: SaveName=ScopeData11
  w_rw : Scope
      settings: SaveName=ScopeData12
  w_rw_Y_0 : Constant  Value=0
  T_rw_Y : Outport
  w_rw_Y : Outport  Port=2
  H_rw_Y : Outport  Port=3
  w_rw_req_Y : Outport  Port=4
  wires:
  T_c_Y/1 -> Product1/1
  Is/1 -> Product1/2, Product2/2, Product3/2
  Product1/1 -> Integrator2/1
  w_rw_Y_0/1 -> Integrator2/2, Integrator3/2
  Integrator2/1 -> Sum/1, w_rw_req_Y/1  "w_rw_required"
  Integrator3/1 -> Sum/2, w_rw_Y/1, w_rw/1, Product3/1
  Sum/1 -> Dead Zone/1
  Gain/1 -> "Saturation max RW rate of change "/1
  Product2/1 -> Integrator3/1
  "Saturation max RW rate of change "/1 -> Product2/1, T_rw_Y/1, T_rw/1
  Spinning Wheel/1(M Inertia Iw) -> Is/1
  Product3/1 -> H_rw_Y/1
  Dead Zone/1 -> Gain/1

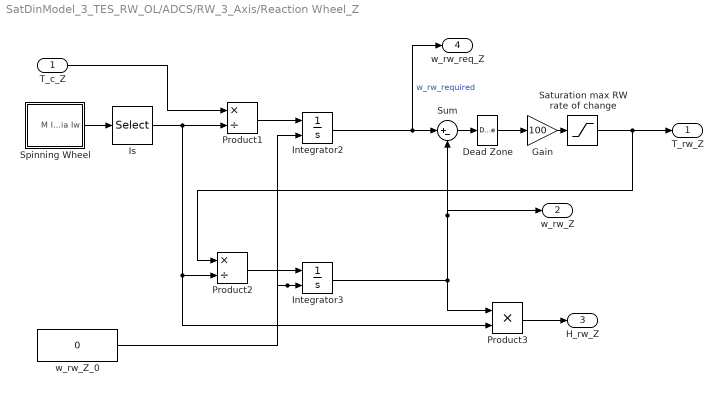
== system SatDinModel_3_TES_RW_OL/ADCS/RW_3_Axis/Reaction Wheel_Z ==
  T_c_Z : Inport
  Dead Zone : DeadZone  SaturateOnIntegerOverflow=on
  Gain : Gain  Gain=100
  Integrator2 : Integrator  InitialConditionSource=external
  Integrator3 : Integrator  InitialConditionSource=external
  Is : Selector  InputPortWidth=3  IndexOptions=Index vector (dialog)  Indices=[1]  OutputSizes=1
  Product1 : Product  Inputs=*/  RndMeth=Zero
  Product2 : Product  Inputs=*/  RndMeth=Zero
  Product3 : Product  RndMeth=Zero
  "Saturation max RW rate of change " : Saturate  UpperLimit=0.0075  LowerLimit=-0.0075
  Spinning Wheel : Subsystem  mask{D=0.1, t=0.01, rho=2850}
      mask prompts: D "diameter"; t "tebal"; rho "density"
  Sum : Sum  Inputs=|+-
  w_rw_Z_0 : Constant  Value=0
  T_rw_Z : Outport
  w_rw_Z : Outport  Port=2
  H_rw_Z : Outport  Port=3
  w_rw_req_Z : Outport  Port=4
  wires:
  T_c_Z/1 -> Product1/1
  Is/1 -> Product1/2, Product2/2, Product3/2
  Product1/1 -> Integrator2/1
  w_rw_Z_0/1 -> Integrator2/2, Integrator3/2
  Integrator2/1 -> Sum/1, w_rw_req_Z/1  "w_rw_required"
  Integrator3/1 -> Sum/2, w_rw_Z/1, Product3/1
  Sum/1 -> Dead Zone/1
  Gain/1 -> "Saturation max RW rate of change "/1
  Product2/1 -> Integrator3/1
  "Saturation max RW rate of change "/1 -> Product2/1, T_rw_Z/1
  Spinning Wheel/1(M Inertia Iw) -> Is/1
  Product3/1 -> H_rw_Z/1
  Dead Zone/1 -> Gain/1

== system SatDinModel_3_TES_RW_OL/Checking/EulerAngles to Others/teta_ZYX to DCM ==
  In2 : Inport
  Create 3x3 Matrix : aerolibutil/Create 3x3 Matrix  SystemSampleTime=-1
  Fcn : Fcn  Expr=cos(u(2))*cos(u(1))
  Fcn1 : Fcn  Expr=cos(u(2))*sin(u(1))
  Fcn2 : Fcn  Expr=-sin(u(2))
  Fcn3 : Fcn  Expr=-cos(u(3))*sin(u(1))+sin(u(3))*sin(u(2))*cos(u(1))
  Fcn4 : Fcn  Expr=cos(u(3))*cos(u(1))+sin(u(3))*sin(u(2))*sin(u(1))
  Fcn5 : Fcn  Expr=sin(u(3))*cos(u(2))
  Fcn6 : Fcn  Expr=sin(u(3))*sin(u(1))+cos(u(3))*sin(u(2))*cos(u(1))
  Fcn7 : Fcn  Expr=-cos(u(1))*sin(u(3))+cos(u(3))*sin(u(2))*sin(u(1))
  Fcn8 : Fcn  Expr=cos(u(3))*cos(u(2))
  Out1 : Outport
  wires:
  Fcn8/1 -> Create 3x3 Matrix/9
  Fcn7/1 -> Create 3x3 Matrix/8
  Fcn6/1 -> Create 3x3 Matrix/7
  Fcn5/1 -> Create 3x3 Matrix/6
  Fcn4/1 -> Create 3x3 Matrix/5
  Fcn3/1 -> Create 3x3 Matrix/4
  Fcn2/1 -> Create 3x3 Matrix/3
  Fcn1/1 -> Create 3x3 Matrix/2
  Fcn/1 -> Create 3x3 Matrix/1
  In2/1 -> Fcn2/1, Fcn3/1, Fcn4/1, Fcn5/1, Fcn6/1, Fcn7/1, Fcn8/1, Fcn1/1, Fcn/1
  Create 3x3 Matrix/1 -> Out1/1

== system SatDinModel_3_TES_RW_OL/Checking/Quaternions to Others/teta_ZYX to DCM ==
  In2 : Inport
  Create 3x3 Matrix : aerolibutil/Create 3x3 Matrix  SystemSampleTime=-1
  Fcn : Fcn  Expr=cos(u(2))*cos(u(1))
  Fcn1 : Fcn  Expr=cos(u(2))*sin(u(1))
  Fcn2 : Fcn  Expr=-sin(u(2))
  Fcn3 : Fcn  Expr=-cos(u(3))*sin(u(1))+sin(u(3))*sin(u(2))*cos(u(1))
  Fcn4 : Fcn  Expr=cos(u(3))*cos(u(1))+sin(u(3))*sin(u(2))*sin(u(1))
  Fcn5 : Fcn  Expr=sin(u(3))*cos(u(2))
  Fcn6 : Fcn  Expr=sin(u(3))*sin(u(1))+cos(u(3))*sin(u(2))*cos(u(1))
  Fcn7 : Fcn  Expr=-cos(u(1))*sin(u(3))+cos(u(3))*sin(u(2))*sin(u(1))
  Fcn8 : Fcn  Expr=cos(u(3))*cos(u(2))
  Out1 : Outport
  wires:
  Fcn8/1 -> Create 3x3 Matrix/9
  Fcn7/1 -> Create 3x3 Matrix/8
  Fcn6/1 -> Create 3x3 Matrix/7
  Fcn5/1 -> Create 3x3 Matrix/6
  Fcn4/1 -> Create 3x3 Matrix/5
  Fcn3/1 -> Create 3x3 Matrix/4
  Fcn2/1 -> Create 3x3 Matrix/3
  Fcn1/1 -> Create 3x3 Matrix/2
  Fcn/1 -> Create 3x3 Matrix/1
  In2/1 -> Fcn2/1, Fcn3/1, Fcn4/1, Fcn5/1, Fcn6/1, Fcn7/1, Fcn8/1, Fcn1/1, Fcn/1
  Create 3x3 Matrix/1 -> Out1/1

== system SatDinModel_3_TES_RW_OL/ADCS/RW_3_Axis/Reaction Wheel_X/Spinning Wheel Kg.m2 ==
  Demux : Demux  Outputs=3
  Moment of Inertia : MATLABFcn  MATLABFcn=momentofinertia_Wheel  Output1D=off
  Mux : Mux  Inputs=3
  Mux1 : Mux  Inputs=3
  db : Constant  Value=rho  VectorParams1D=off
  diameter : Constant  Value=D  VectorParams1D=off
  tebal : Constant  Value=t  VectorParams1D=off
  M Inertia Iw : Outport
  wires:
  db/1 -> Mux/1
  diameter/1 -> Mux/2
  tebal/1 -> Mux/3
  Mux/1 -> Moment of Inertia/1
  Demux/1 -> Mux1/1
  Demux/2 -> Mux1/2
  Demux/3 -> Mux1/3
  Moment of Inertia/1 -> Demux/1
  Mux1/1 -> M Inertia Iw/1

== system SatDinModel_3_TES_RW_OL/ADCS/RW_3_Axis/Reaction Wheel_Y/Spinning Wheel ==
  Demux : Demux  Outputs=3
  Moment of Inertia : MATLABFcn  MATLABFcn=momentofinertia_Wheel  Output1D=off
  Mux : Mux  Inputs=3
  Mux1 : Mux  Inputs=3
  db : Constant  Value=rho  VectorParams1D=off
  diameter : Constant  Value=D  VectorParams1D=off
  tebal : Constant  Value=t  VectorParams1D=off
  M Inertia Iw : Outport
  wires:
  db/1 -> Mux/1
  diameter/1 -> Mux/2
  tebal/1 -> Mux/3
  Mux/1 -> Moment of Inertia/1
  Demux/1 -> Mux1/1
  Demux/2 -> Mux1/2
  Demux/3 -> Mux1/3
  Moment of Inertia/1 -> Demux/1
  Mux1/1 -> M Inertia Iw/1

== system SatDinModel_3_TES_RW_OL/ADCS/RW_3_Axis/Reaction Wheel_Z/Spinning Wheel ==
  Demux : Demux  Outputs=3
  Moment of Inertia : MATLABFcn  MATLABFcn=momentofinertia_Wheel  Output1D=off
  Mux : Mux  Inputs=3
  Mux1 : Mux  Inputs=3
  db : Constant  Value=rho  VectorParams1D=off
  diameter : Constant  Value=D  VectorParams1D=off
  tebal : Constant  Value=t  VectorParams1D=off
  M Inertia Iw : Outport
  wires:
  db/1 -> Mux/1
  diameter/1 -> Mux/2
  tebal/1 -> Mux/3
  Mux/1 -> Moment of Inertia/1
  Demux/1 -> Mux1/1
  Demux/2 -> Mux1/2
  Demux/3 -> Mux1/3
  Moment of Inertia/1 -> Demux/1
  Mux1/1 -> M Inertia Iw/1

== matlab function TIME/Embedded MATLAB Function ==
  data: jd input double; y output double
function y = fcn(jd)
%#eml

 % ----------------- find year and days of the year ---------------
     temp   = jd-2415019.5+1721044.5+14;
     tu     = temp / 365.25;
     year   = 1900 + floor( tu );
     leapyrs= floor( ( year-1901 )*0.25 );
%     days   = temp - ((year-1900)*365.0 + leapyrs ) + 0.00000000001; % nudge by 8.64x10-7 sec to get even outputs
     days   = temp - ((year-1900)*365.0 + leapyrs );

     % ------------ check for case of beginning of a year -------------
     if days < 1.0
         year   = year - 1;
         leapyrs= floor( ( year-1901 )*0.25 );
         days   = temp - ((year-1900)*365.0 + leapyrs );
       end

     % ------------------- find remaining data  -----------------------
     
     % --------------- set up array of days in month  --------------
     lmonth=[31;28;31;30;31;30;31;31;30;31;30;31];
          
     dayofyr= floor(days );

        % ----------------- find month and day of month ---------------
        if modulo(year-1900,4) == 0
            lmonth(2)= 29;
          end

        i= 1;
        inttemp= 0;
        while ( dayofyr > inttemp + lmonth(i) ) & ( i < 12 )
            inttemp= inttemp + lmonth(i);
            i= i+1;
          end

        mon= i;
        day= dayofyr - inttemp;

        % ----------------- find hours minutes and seconds ------------
        temp= (days - dayofyr )*24.0;
        hr  = fix( temp );
        temp= (temp-hr) * 60.0;
        min = fix( temp );
        sec = (temp-min) * 60.0;
%     sec= sec - 0.00000086400;


y = [year;mon;day;hr;min;sec];
